simulink model "Pendulum_CAD_Control2293_LoopShaping_2018A"  (R2018a)
settings: Solver=ode15s  StartTime=0.0  StopTime=30  MaxStep=1e-3  RelTol=1e-3  EnableMultiTasking=on
PreLoadFcn:
  | RotaryPendulum_PARAM
values from neighbouring files (symbols this model uses):
  Kl1 = 1/db2mag(40)    [CalculoParametrosV2.m]
  Kl2 = 1/db2mag(-12)    [CalculoParametrosV2.m]
  s = tf('s')    [CalculoParametrosV2.m]
undefined symbols (not defined in the file or in its folder): controller_on_off, K2, length_base, length_vert_cylinder, radius_vert_cylinder, X, Y, Z
libraries: sm_lib x48, nesl_utility x6, fl_lib x4, cstblocks x2, simulink x1, aerolibanimutils x1
(part 1 of 2)
settings Model: ParamWorkspaceSource=ReferencedWorkspace  TunableVars=controller_on_off,friction_on_off  TunableVarsStorageClass=ExportedGlobal,ExportedGlobal  TunableVarsTypeQualifier=,  Creator=smalack  LastModifiedBy=Marcelo
settings DataIOCC: LimitDataPoints=on  SaveFormat=Array
settings OptimizationCC: DefaultParameterBehavior=Inlined  LifeSpan=inf
settings DebuggingCC: SFUnexpectedBacktrackingDiag=warning  SFNoUnconditionalDefaultTransitionDiag=warning  SFExecutionAtInitializationDiag=none
settings HardwareCC: ProdBitPerPointer=32  ProdBitPerSizeT=32  ProdBitPerPtrDiffT=32  ProdLargestAtomicFloat=None  ProdIntDivRoundTo=Undefined  ProdEndianess=Unspecified  ProdWordSize=32  ProdHWDeviceType=32-bit Generic
settings ModelReferenceCC: PropagateSignalLabelsOutOfModel=off
settings CodeAppCC: StateflowObjectComments=on
settings GRTTargetCC: TargetLangStandard=C89/C90 (ANSI)
settings ConfigComp: CovMetricSettings=dw  CovHtmlReporting=on  CovSaveCumulativeToWorkspaceVar=on  CovSaveSingleToWorkspaceVar=on  CovExternalEMLEnable=off
settings SimscapeCC: SimscapeNormalizeSystem=off
settings ConfigurationSet: Description=SimMechanics 2G
settings ExplorerConfigSet: InternalSimMechanicsExplorerSettings="<ExplorerConfiguration><canonicalview>default</canonicalview><AnimationSetting><BasePlaybackSpeed>1.0</BasePlaybackSpeed><PlaybackSpeedFactor>1.0</PlaybackSpeedFactor></AnimationSetting><TilePanel><TileInfo><Tiles Columns=\"1\" Count=\"1\" Rows=\"1\"><Column Weight=\"1\"/><Row Weight=\"1\"/><Tile Height=\"1\" Width=\"1\" X=\"0\" Y=\"0\"/></Tiles></TileInfo><SceneInfo><SceneViewer><BGColor><R>0.866666674613952637</R><G>0.866666674613952637</G><B>0.866666674613952637</B></BGColor><Camera><DoPerspective>off</DoPerspective><Position><X>0.54567988539648471</X><Y>0.116966334833298546</Y><Z>0.211463718228743575</Z></Position><Center><X>0.0539563667929072593</X><Y>0.0515860641109495213</Y><Z>0.183072620253275059</Z></Center><Up><X>-0.0571571554031080065</X><Y>-0.00365517739132248387</Y><Z>0.998358502375005452</Z></Up><ViewLimDist>1</ViewLimDist><YLim>0.200635310715059134</YLim><XLim>0.295379762997170392</XLim></Camera></SceneViewer></SceneInfo></TilePanel><MechEditorPanel><Cameras/><GfxPanelCameraMap/><VideoCreator><PlaybackSpeedRatio>1.0</PlaybackSpeedRatio><FrameRate>30</FrameRate><VideoFormat>MPEG-4</VideoFormat><FrameSize>auto</FrameSize></VideoCreator></MechEditorPanel></ExplorerConfiguration>"

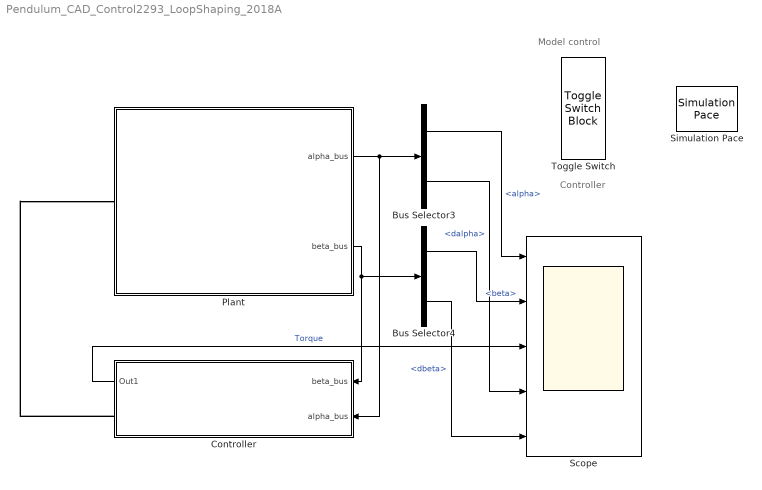
== system Pendulum_CAD_Control2293_LoopShaping_2018A ==
  note: Model control
  note: Controller
  Bus Selector3 : BusSelector  OutputSignals=alpha,dalpha
  Bus Selector4 : BusSelector  OutputSignals=beta,dbeta
  Controller : Subsystem  mask{energy_gain=0.36, switch_angle=30, alpha=K2(1), alpha_dot=K2(3), beta=K2(2), beta_dot=K2(4)}
      mask prompts: energy_gain "energy control gain [-]"; switch_angle "switch angle [deg]"; alpha "alpha [-]"; alpha_dot "alpha_dot [-]"; beta "beta [-]"; beta_dot "beta_dot [-]"
      mask DialogControl Container20 Prompt: SwingUp Control
      mask DialogControl Container17 Prompt: SwingUp to StayUp
      mask DialogControl Container10 Prompt: StayUp Control
      mask Display:
      | disp('{\itcontrol variable=}  k\timesE\timessign(\partial{\beta}/\partial{t} \times cos(\beta))', 'texmode','on')
      | port_label('input', 2, 'alpha_bus')
      | port_label('input', 1, 'beta_bus')
  Plant : Subsystem
      mask Display:
      | image('overall.JPG')
      | port_label('lconn',1,'torque');
      | port_label('output', 1, 'alpha_bus')
      | port_label('output', 2, 'beta_bus')
  Scope : Scope  NumInputPorts=5
  Simulation Pace : aerolibanimutils/Simulation Pace  SimulationPace=1  SleepMode=MATLAB Thread  OutputPaceError=off  SampleTime=1/30
      settings: AttributesFormatString=%<SimulationPace> sec/sec
  Toggle Switch : ToggleSwitchBlock  WebBlockId=671
      settings: Values={{'Off', 'On'}, [0 1]}
  wires:
  Plant/2(beta_bus) -> Controller/1(beta_bus), Bus Selector4/1
  Plant/1(alpha_bus) -> Bus Selector3/1, Controller/2(alpha_bus)
  Bus Selector3/1 -> Scope/1  "<alpha>"
  Bus Selector4/1 -> Scope/2  "<beta>"
  Bus Selector3/2 -> Scope/4  "<dalpha>"
  Bus Selector4/2 -> Scope/5  "<dbeta>"
  Controller/1(Out1) -> Scope/3  "Torque"
  connections:
  Controller/RConn1 -- Plant/LConn1

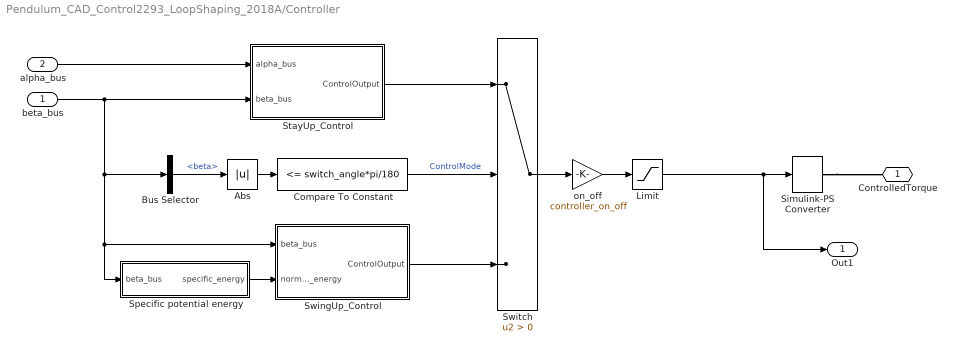
== system Pendulum_CAD_Control2293_LoopShaping_2018A/Controller ==
  beta_bus : Inport
  alpha_bus : Inport  Port=2
  Abs : Abs
  Bus Selector : BusSelector  OutputSignals=beta
  Compare To Constant : simulink/Logic and Bit Operations/Compare To Constant  relop=<=  const=switch_angle*pi/180  OutDataTypeStr=boolean
  Limit : Saturate  UpperLimit=0.1e3  LowerLimit=-0.1e3
  Simulink-PS Converter : nesl_utility/Simulink-PS Converter  PhysicalDomain=network_engine_domain  SubClassName=ps_input  LeftPortType=input  RightPortType=output  PseudoPeriodic=off  Frequencies=[]  NoiseDistribution=none  NoiseParameters=[]  Unit=N*mm  AffineConversion=off  FilteringAndDerivatives=zero  SimscapeFilterOrder=1  InputFilterTimeConstant=0.001  UdotUserProvided=1
  Specific potential energy : Subsystem
  StayUp_Control : Subsystem
  SwingUp_Control : Subsystem  mask{Gain=energy_gain}
      mask prompts: Gain "Simulink:blkprm_prompts:GainGain"
      mask TypeOptions Gain: Gain/Gain
      mask DialogControl Gain Prompt: Gain:
  Switch : Switch  Criteria=u2 > Threshold
  on_off : Gain  Gain=controller_on_off
  ControlledTorque : PMIOPort  Side=Right
  Out1 : Outport  VectorParamsAs1DForOutWhenUnconnected=off
  wires:
  alpha_bus/1 -> StayUp_Control/1(alpha_bus)
  Compare To Constant/1 -> Switch/2  "ControlMode"
  Abs/1 -> Compare To Constant/1
  Bus Selector/1 -> Abs/1  "<beta>"
  beta_bus/1 -> StayUp_Control/2(beta_bus), SwingUp_Control/1(beta_bus), Specific potential energy/1(beta_bus), Bus Selector/1
  SwingUp_Control/1(ControlOutput) -> Switch/3
  Switch/1 -> on_off/1
  on_off/1 -> Limit/1
  Specific potential energy/1(specific_energy) -> SwingUp_Control/2(normalized_energy)
  Limit/1 -> Out1/1, Simulink-PS Converter/1
  StayUp_Control/1(ControlOutput) -> Switch/1
  connections:
  Simulink-PS Converter/RConn1 -- ControlledTorque/RConn1

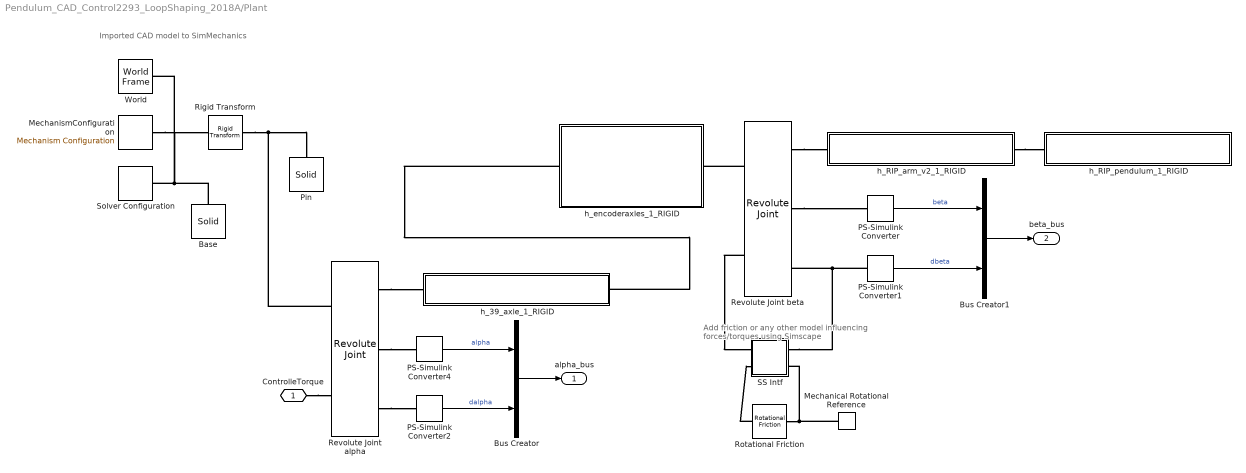
== system Pendulum_CAD_Control2293_LoopShaping_2018A/Plant ==
  note: Imported CAD model to SimMechanics
  note: Add friction or any other model
      | influencing forces/torques using Simscape
  Base : sm_lib/Body Elements/Solid  GraphicAmbientColor=[0.15 0.15 0.15 1.0]  BasedOnType=Density  CenterOfMass=[0 0 0]  CenterOfMassUnits=m  GraphicDiffuseColor=[0.4 0.4 0.4]  CylinderLength=length_base  CylinderLengthUnits=m  CylinderRadius=radius_base  CylinderRadiusUnits=m  Density=2700  DensityUnits=kg/(m^3)  DoExposeReferenceFrame=on  GraphicEmissiveColor=[0.0 0.0 0.0 1.0]  ExportEntireGeometry=off  SerializedFrames=<Frames/>  MarkerShape=Sphere  MarkerSize=10  GraphicType=FromGeometry  InertiaType=CalculateFromGeometry  Mass=1  MassUnits=kg  MomentsOfInertia=[1 1 1]  MomentsOfInertiaUnits=kg*m^2  GraphicOpacity=1.0  ProductsOfInertia=[0 0 0]  ProductsOfInertiaUnits=kg*m^2  GraphicShininess=75  GraphicSpecularColor=[0.5 0.5 0.5 1.0]  GraphicVisPropType=SimpleVisualProperties  GeometryShape=Cylinder
  Bus Creator : BusCreator  Inputs=2
  Bus Creator1 : BusCreator  Inputs=2
  Mechanical Rotational Reference : fl_lib/Mechanical/Rotational Elements/Mechanical Rotational Reference
  MechanismConfiguration : sm_lib/Utilities/Mechanism Configuration  UniformGravity=Constant  GravityVector=[0 0 -9.81]  GravityUnits=m/s^2  LinearizationDelta=0.001
  PS-Simulink Converter : nesl_utility/PS-Simulink Converter  PhysicalDomain=network_engine_domain  SubClassName=ps_output  LeftPortType=input  RightPortType=output  PseudoPeriodic=off  Frequencies=[]  Unit=rad  AffineConversion=off
  PS-Simulink Converter1 : nesl_utility/PS-Simulink Converter  PhysicalDomain=network_engine_domain  SubClassName=ps_output  LeftPortType=input  RightPortType=output  PseudoPeriodic=off  Frequencies=[]  Unit=rad/s  AffineConversion=off
  PS-Simulink Converter2 : nesl_utility/PS-Simulink Converter  PhysicalDomain=network_engine_domain  SubClassName=ps_output  LeftPortType=input  RightPortType=output  PseudoPeriodic=off  Frequencies=[]  Unit=rad/s  AffineConversion=off
  PS-Simulink Converter4 : nesl_utility/PS-Simulink Converter  PhysicalDomain=network_engine_domain  SubClassName=ps_output  LeftPortType=input  RightPortType=output  PseudoPeriodic=off  Frequencies=[]  Unit=rad  AffineConversion=off
  Pin : sm_lib/Body Elements/Solid  GraphicAmbientColor=[0.15 0.15 0.15 1.0]  BasedOnType=Density  CenterOfMass=[0 0 0]  CenterOfMassUnits=m  GraphicDiffuseColor=[0.8 0.6 1.0]  CylinderLength=length_vert_cylinder  CylinderLengthUnits=m  CylinderRadius=radius_vert_cylinder/2  CylinderRadiusUnits=m  Density=2700  DensityUnits=kg/(m^3)  DoExposeReferenceFrame=on  GraphicEmissiveColor=[0.0 0.0 0.0 1.0]  ExportEntireGeometry=off  SerializedFrames=<Frames/>  MarkerShape=Sphere  MarkerSize=10  GraphicType=FromGeometry  InertiaType=CalculateFromGeometry  Mass=1  MassUnits=kg  MomentsOfInertia=[1 1 1]  MomentsOfInertiaUnits=kg*m^2  GraphicOpacity=.5  ProductsOfInertia=[0 0 0]  ProductsOfInertiaUnits=kg*m^2  GraphicShininess=75  GraphicSpecularColor=[0.5 0.5 0.5 1.0]  GraphicVisPropType=SimpleVisualProperties  GeometryShape=Cylinder
  Revolute Joint alpha : sm_lib/Joints/Revolute Joint  JointMode=Normal  SenseConstraintForce=off  SenseConstraintForceX=off  SenseConstraintForceY=off  SenseConstraintForceZ=off  SenseConstraintTorque=off  SenseConstraintTorqueX=off  SenseConstraintTorqueY=off  SenseConstraintTorqueZ=off  SenseTotalForce=off  SenseTotalForceX=off  SenseTotalForceY=off  SenseTotalForceZ=off  SenseTotalTorque=off  SenseTotalTorqueX=off  SenseTotalTorqueY=off  SenseTotalTorqueZ=off  CompositeWrenchDir=FollowerOnBase  CompositeWrenchFrame=BaseFrame  EquilibriumPosition=0  EquilibriumPositionUnits=deg  SpringStiffness=1e-7  SpringStiffnessUnits=N*m/deg  DampingCoefficient=1e-6  DampingCoefficientUnits=N*m/(deg/s)  TorqueActuationMode=InputTorque  MotionActuationMode=ComputedMotion  SensePosition=on  SenseVelocity=on  SenseAcceleration=off  SenseTorqueForce=off  SenseLowerLimitTorqueForce=off  SenseUpperLimitTorqueForce=off  LowerLimitSpecify=off  LowerLimitBound=-90  LowerLimitBoundUnits=deg  LowerLimitStiffness=1e4  LowerLimitStiffnessUnits=N*m/deg  LowerLimitDamping=10  LowerLimitDampingUnits=N*m/(deg/s)  LowerLimitTransitionRegionWidth=0.1  LowerLimitTransitionRegionWidthUnits=deg  UpperLimitSpecify=off  UpperLimitBound=90  UpperLimitBoundUnits=deg  UpperLimitStiffness=1e4  UpperLimitStiffnessUnits=N*m/deg  UpperLimitDamping=10  UpperLimitDampingUnits=N*m/(deg/s)  UpperLimitTransitionRegionWidth=0.1  UpperLimitTransitionRegionWidthUnits=deg  PositionTargetSpecify=off  PositionTargetPriority=High  PositionTargetValue=pi  PositionTargetValueUnits=rad  VelocityTargetSpecify=off  VelocityTargetPriority=High  VelocityTargetValue=0  VelocityTargetValueUnits=deg/s
  Revolute Joint beta : sm_lib/Joints/Revolute Joint  JointMode=Normal  SenseConstraintForce=off  SenseConstraintForceX=off  SenseConstraintForceY=off  SenseConstraintForceZ=off  SenseConstraintTorque=off  SenseConstraintTorqueX=off  SenseConstraintTorqueY=off  SenseConstraintTorqueZ=off  SenseTotalForce=off  SenseTotalForceX=off  SenseTotalForceY=off  SenseTotalForceZ=off  SenseTotalTorque=off  SenseTotalTorqueX=off  SenseTotalTorqueY=off  SenseTotalTorqueZ=off  CompositeWrenchDir=FollowerOnBase  CompositeWrenchFrame=BaseFrame  EquilibriumPosition=0  EquilibriumPositionUnits=rad  SpringStiffness=0  SpringStiffnessUnits=m*N/rad  DampingCoefficient=0  DampingCoefficientUnits=m*s*N/rad  TorqueActuationMode=InputTorque  MotionActuationMode=ComputedMotion  SensePosition=on  SenseVelocity=on  SenseAcceleration=off  SenseTorqueForce=off  SenseLowerLimitTorqueForce=off  SenseUpperLimitTorqueForce=off  LowerLimitSpecify=off  LowerLimitBound=-90  LowerLimitBoundUnits=deg  LowerLimitStiffness=1e4  LowerLimitStiffnessUnits=N*m/deg  LowerLimitDamping=10  LowerLimitDampingUnits=N*m/(deg/s)  LowerLimitTransitionRegionWidth=0.1  LowerLimitTransitionRegionWidthUnits=deg  UpperLimitSpecify=off  UpperLimitBound=90  UpperLimitBoundUnits=deg  UpperLimitStiffness=1e4  UpperLimitStiffnessUnits=N*m/deg  UpperLimitDamping=10  UpperLimitDampingUnits=N*m/(deg/s)  UpperLimitTransitionRegionWidth=0.1  UpperLimitTransitionRegionWidthUnits=deg  PositionTargetSpecify=on  PositionTargetPriority=Low  PositionTargetValue=180  PositionTargetValueUnits=deg  VelocityTargetSpecify=on  VelocityTargetPriority=High  VelocityTargetValue=0  VelocityTargetValueUnits=deg/s
  Rigid Transform : sm_lib/Frames and Transforms/Rigid Transform  TranslationMethod=StandardAxis  TranslationStandardOffset=length_base/2+length_vert_cylinder/2  TranslationLengthUnit=m  TranslationStandardAxis=+Z  TranslationCartesianOffset=[0 0 0]  TranslationROffset=0  TranslationROffsetUnits=m  TranslationZOffset=0  TranslationZOffsetUnits=m  TranslationThetaOffset=0  TranslationThetaOffsetUnits=deg  RotationMethod=None  RotationAngleUnits=deg  RotationStandardAxis=+Z  RotationAngle=0.0  RotationArbitraryAxis=[0 0 1]  FollAlignAxisA=+X  BaseAlignAxisA=+Y  FollAlignAxisB=+Y  BaseAlignAxisB=+Z  RotationSequenceAxes=FollowerAxes  RotationSequence=XYX  RotationSequenceAngles=[0 0 0]  RotationSequenceAnglesUnits=deg  RotationMatrix=[1 0 0; 0 1 0; 0 0 1]
  Rotational Friction : fl_lib/Mechanical/Rotational Elements/Rotational Friction  brkwy_trq=0.0004 mN*m  brkwy_vel=0.12128 rad/s  Col_trq=0.0002 mN*m  visc_coef=0.001 m*s*mN/rad  w_specify=off  w_priority=High  w=0 rad/s  w_nominal_specify=off  w_nominal_unit=rad/s  w_nominal_value=1  t_specify=off  t_priority=High  t=0 N*m  t_nominal_specify=off  t_nominal_unit=N*m  t_nominal_value=1
  SS Intf : Subsystem
  Solver Configuration : nesl_utility/Solver Configuration  PhysicalDomain=network_engine_domain  SubClassName=solver  LeftPortType=input  RightPortType=generic  Tones=[]  Harmonics=[]  SimulateNoise=off  Profile=off  UseLocalSampling=off  EnableSwitchedLinearOptims=on  FrequencyDomain=off  UseCCode=off  RelTol=0.001  AbsTol=1e-06  MinStep=1e-09  ToWorkspace=off  RevertToSquareIcSolve=off  NumHomotopyIterations=100  PhasorMode=off  PhasorModeNumHarmonics=1  DoDC=off  ResidualTolerance=1e-09  UseLocalSolver=off  LocalSolverChoice=NE_BACKWARD_EULER_ADVANCER  LocalSolverSampleTime=1e-3  DoFixedCost=off  MaxNonlinIter=3  MaxModeIter=2  LinearAlgebra=Sparse  EquationFormulation=NE_TIME_EF  DelaysMemoryBudget=1024  AutomaticFiltering=on  FilteringTimeConstant=0.001  PartitionStorageMethod=AS_NEEDED  PartitionMemoryBudget=1024  PartitionMethod=FAST
  World : sm_lib/Frames and Transforms/World Frame
  h_39_axle_1_RIGID : Subsystem
      mask Display:
      | image('h_39_axle_1_RIGID.JPG')
      | port_label('lconn',1,'B');
      | port_label('rconn',1,'R');
  h_RIP_arm_v2_1_RIGID : Subsystem
      mask Display:
      | image('h_RIP_arm_v2_1_RIGID.JPG');
      | port_label('lconn',1,'B');
      | port_label('rconn',1,'R');
  h_RIP_pendulum_1_RIGID : Subsystem
      mask Display: image('h_RIP_pendulum_1_RIGID.JPG');
  h_encoderaxles_1_RIGID : Subsystem
      mask Display:
      | image('h_encoderaxles_1_RIGID.JPG');
      | port_label('lconn',1,'B');
      | port_label('rconn',1,'R');
  ControlleTorque : PMIOPort  Side=Left
  alpha_bus : Outport  VectorParamsAs1DForOutWhenUnconnected=off
  beta_bus : Outport  Port=2  VectorParamsAs1DForOutWhenUnconnected=off
  wires:
  Bus Creator/1 -> alpha_bus/1
  Bus Creator1/1 -> beta_bus/1
  PS-Simulink Converter/1 -> Bus Creator1/1  "beta"
  PS-Simulink Converter4/1 -> Bus Creator/1  "alpha"
  PS-Simulink Converter2/1 -> Bus Creator/2  "dalpha"
  PS-Simulink Converter1/1 -> Bus Creator1/2  "dbeta"
  connections:
  Rotational Friction/LConn1 -- SS Intf/RConn2
  Revolute Joint beta/RConn1 -- h_RIP_arm_v2_1_RIGID/LConn1
  Rotational Friction/RConn1 -- Mechanical Rotational Reference/LConn1 -- SS Intf/LConn2
  Revolute Joint alpha/RConn1 -- h_39_axle_1_RIGID/LConn1
  PS-Simulink Converter1/LConn1 -- SS Intf/LConn1 -- Revolute Joint beta/RConn3
  Base/RConn1 -- Rigid Transform/LConn1 -- MechanismConfiguration/RConn1 -- World/RConn1 -- Solver Configuration/RConn1
  Revolute Joint alpha/RConn3 -- PS-Simulink Converter2/LConn1
  h_encoderaxles_1_RIGID/LConn1 -- h_39_axle_1_RIGID/RConn1
  h_RIP_arm_v2_1_RIGID/RConn1 -- h_RIP_pendulum_1_RIGID/LConn1
  Revolute Joint beta/LConn1 -- h_encoderaxles_1_RIGID/RConn1
  Revolute Joint beta/LConn2 -- SS Intf/RConn1
  Revolute Joint alpha/RConn2 -- PS-Simulink Converter4/LConn1
  Revolute Joint beta/RConn2 -- PS-Simulink Converter/LConn1
  ControlleTorque/RConn1 -- Revolute Joint alpha/LConn2
  Rigid Transform/RConn1 -- Revolute Joint alpha/LConn1 -- Pin/RConn1

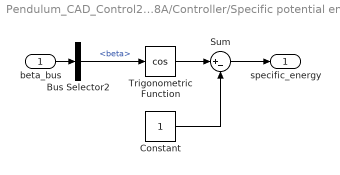
== system Pendulum_CAD_Control2293_LoopShaping_2018A/Controller/Specific potential energy ==
  beta_bus : Inport
  Bus Selector2 : BusSelector  OutputSignals=beta
  Constant : Constant
  Sum : Sum  Inputs=|+-
  Trigonometric Function : Trigonometry  Operator=cos
  specific_energy : Outport  VectorParamsAs1DForOutWhenUnconnected=off
  wires:
  Constant/1 -> Sum/2
  Trigonometric Function/1 -> Sum/1
  Sum/1 -> specific_energy/1
  Bus Selector2/1 -> Trigonometric Function/1  "<beta>"
  beta_bus/1 -> Bus Selector2/1

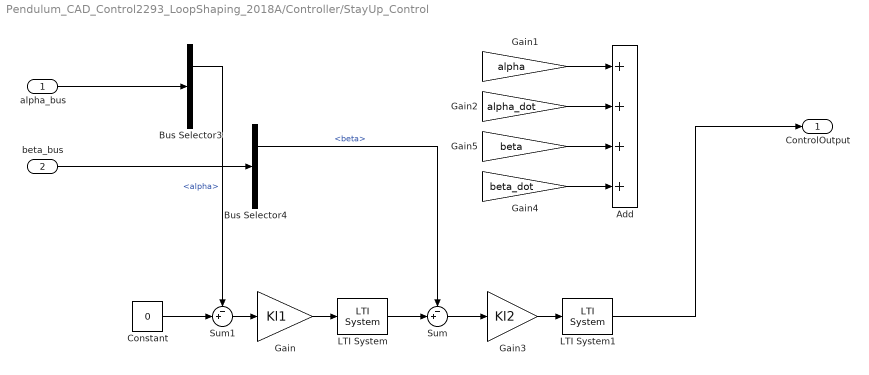
== system Pendulum_CAD_Control2293_LoopShaping_2018A/Controller/StayUp_Control ==
  alpha_bus : Inport
  beta_bus : Inport  Port=2
  Add : Sum  Inputs=++++
  Bus Selector3 : BusSelector  OutputSignals=alpha,dalpha
  Bus Selector4 : BusSelector  OutputSignals=beta,dbeta
  Constant : Constant  Value=0
  Gain : Gain  Gain=Kl1
  Gain1 : Gain  Gain=alpha
  Gain2 : Gain  Gain=alpha_dot
  Gain3 : Gain  Gain=Kl2
  Gain4 : Gain  Gain=beta_dot
  Gain5 : Gain  Gain=beta
  LTI System : cstblocks/LTI System  sys=C1  IC=[]
  LTI System1 : cstblocks/LTI System  sys=C2  IC=[]
  Sum : Sum  Inputs=-+|
  Sum1 : Sum  Inputs=-+|
  ControlOutput : Outport  VectorParamsAs1DForOutWhenUnconnected=off
  wires:
  alpha_bus/1 -> Bus Selector3/1
  Gain5/1 -> Add/3
  Gain1/1 -> Add/1
  Gain4/1 -> Add/4
  beta_bus/1 -> Bus Selector4/1
  Gain2/1 -> Add/2
  Bus Selector3/1 -> Sum1/1  "<alpha>"
  Constant/1 -> Sum1/2
  LTI System1/1 -> ControlOutput/1
  Gain/1 -> LTI System/1
  Sum1/1 -> Gain/1
  Gain3/1 -> LTI System1/1
  Sum/1 -> Gain3/1
  Bus Selector4/1 -> Sum/1  "<beta>"
  LTI System/1 -> Sum/2

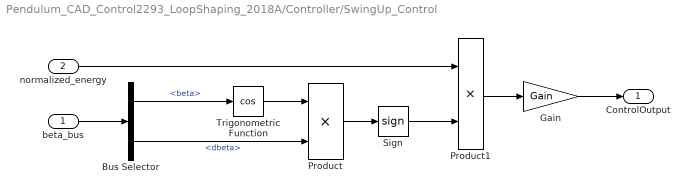
== system Pendulum_CAD_Control2293_LoopShaping_2018A/Controller/SwingUp_Control ==
  beta_bus : Inport
  normalized_energy : Inport  Port=2
  Bus Selector : BusSelector  OutputSignals=beta,dbeta
  Gain : Gain  Gain=Gain
  Product : Product
  Product1 : Product
  Sign : Signum
  Trigonometric Function : Trigonometry  Operator=cos
  ControlOutput : Outport  VectorParamsAs1DForOutWhenUnconnected=off
  wires:
  Product/1 -> Sign/1
  Trigonometric Function/1 -> Product/1
  Gain/1 -> ControlOutput/1
  Sign/1 -> Product1/2
  Product1/1 -> Gain/1
  normalized_energy/1 -> Product1/1
  beta_bus/1 -> Bus Selector/1
  Bus Selector/1 -> Trigonometric Function/1  "<beta>"
  Bus Selector/2 -> Product/2  "<dbeta>"

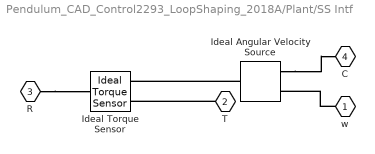
== system Pendulum_CAD_Control2293_LoopShaping_2018A/Plant/SS Intf ==
  Ideal Angular Velocity Source : fl_lib/Mechanical/Mechanical Sources/Ideal Angular Velocity Source
  Ideal Torque Sensor : fl_lib/Mechanical/Mechanical Sensors/Ideal Torque Sensor
  w : PMIOPort  Side=Left
  T : PMIOPort  Port=2  Side=Right
  R : PMIOPort  Port=3  Side=Right
  C : PMIOPort  Port=4  Side=Left
  connections:
  w/RConn1 -- Ideal Angular Velocity Source/RConn1
  R/RConn1 -- Ideal Torque Sensor/LConn1
  Ideal Angular Velocity Source/RConn2 -- C/RConn1
  Ideal Angular Velocity Source/LConn1 -- Ideal Torque Sensor/RConn1
  T/RConn1 -- Ideal Torque Sensor/RConn2

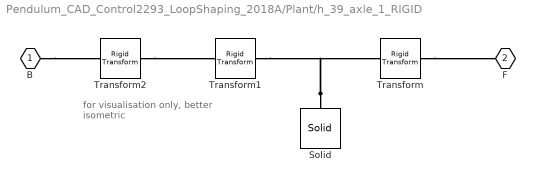
== system Pendulum_CAD_Control2293_LoopShaping_2018A/Plant/h_39_axle_1_RIGID ==
  note: for visualisation only,
      | better isometric
  Solid : sm_lib/Body Elements/Solid  ExtGeomFileName=h_39_axle_Default_sldprt.STL  UnitType=Custom  ExtGeomFileUnits=mm  StepReaderType=HEX  ExportConvexHullGeometry=off  InertiaType=Custom  Mass=0.00052672018519800228  MassUnits=kg  CenterOfMass=[0 0 0]  CenterOfMassUnits=mm  MomentsOfInertia=[0.0012508560304239273 0.066771141817072402 0.066771141817072402]  MomentsOfInertiaUnits=kg*mm^2  ProductsOfInertia=[0 0 0]  ProductsOfInertiaUnits=kg*mm^2  BasedOnType=Density  Density=1000  DensityUnits=kg/(m^3)  DoExposeReferenceFrame=on  SerializedFrames=<Frames/>  GraphicType=FromGeometry  MarkerShape=Sphere  MarkerSize=10  MarkerSizeUnits=m  GraphicVisPropType=SimpleVisualProperties  GraphicDiffuseColor=[0.4 0.4 0.4]  GraphicSpecularColor=[0.5 0.5 0.5 1.0]  GraphicAmbientColor=[0.15 0.15 0.15 1.0]  GraphicEmissiveColor=[0.0 0.0 0.0 1.0]  GraphicShininess=75  GraphicOpacity=1  GeometryShape=FromFile
  Transform : sm_lib/Frames and Transforms/Rigid Transform  TranslationMethod=Cartesian  TranslationStandardOffset=0  TranslationLengthUnit=mm  TranslationStandardAxis=+Z  TranslationCartesianOffset=[19.5 1.2534832698893993 1.25543121904946712 ]  TranslationROffset=0  TranslationROffsetUnits=m  TranslationZOffset=0  TranslationZOffsetUnits=m  TranslationThetaOffset=0  TranslationThetaOffsetUnits=deg  RotationMethod=StandardAxis  RotationAngleUnits=rad  RotationStandardAxis=-Y  RotationAngle=pi/2  RotationArbitraryAxis=[0.70549464967288755 0.067487766045881178 -0.70549464967288456]  FollAlignAxisA=+X  BaseAlignAxisA=+Y  FollAlignAxisB=+Y  BaseAlignAxisB=+Z  RotationSequenceAxes=FollowerAxes  RotationSequence=XYX  RotationSequenceAngles=[0 0 0]  RotationSequenceAnglesUnits=deg  RotationMatrix=[1 0 0; 0 1 0; 0 0 1]
  Transform1 : sm_lib/Frames and Transforms/Rigid Transform  TranslationMethod=Cartesian  TranslationStandardOffset=0  TranslationLengthUnit=mm  TranslationStandardAxis=+Z  TranslationCartesianOffset=[0 0 19.5]  TranslationROffset=0  TranslationROffsetUnits=m  TranslationZOffset=0  TranslationZOffsetUnits=m  TranslationThetaOffset=0  TranslationThetaOffsetUnits=deg  RotationMethod=StandardAxis  RotationAngleUnits=rad  RotationStandardAxis=-Y  RotationAngle=pi/2  RotationArbitraryAxis=[0.70549464967288755 0.067487766045881178 -0.70549464967288456]  FollAlignAxisA=+X  BaseAlignAxisA=+Y  FollAlignAxisB=+Y  BaseAlignAxisB=+Z  RotationSequenceAxes=FollowerAxes  RotationSequence=XYX  RotationSequenceAngles=[0 0 0]  RotationSequenceAnglesUnits=deg  RotationMatrix=[1 0 0; 0 1 0; 0 0 1]
  Transform2 : sm_lib/Frames and Transforms/Rigid Transform  TranslationMethod=Cartesian  TranslationStandardOffset=0  TranslationLengthUnit=mm  TranslationStandardAxis=+Z  TranslationCartesianOffset=[0 0 19.5]  TranslationROffset=0  TranslationROffsetUnits=m  TranslationZOffset=0  TranslationZOffsetUnits=m  TranslationThetaOffset=0  TranslationThetaOffsetUnits=deg  RotationMethod=StandardAxis  RotationAngleUnits=rad  RotationStandardAxis=+Z  RotationAngle=pi  RotationArbitraryAxis=[0.70549464967288755 0.067487766045881178 -0.70549464967288456]  FollAlignAxisA=+X  BaseAlignAxisA=+Y  FollAlignAxisB=+Y  BaseAlignAxisB=+Z  RotationSequenceAxes=FollowerAxes  RotationSequence=XYX  RotationSequenceAngles=[0 0 0]  RotationSequenceAnglesUnits=deg  RotationMatrix=[1 0 0; 0 1 0; 0 0 1]
  B : PMIOPort  Side=Left
  F : PMIOPort  Port=2  Side=Right
  connections:
  Solid/RConn1 -- Transform1/RConn1 -- Transform/LConn1
  Transform/RConn1 -- F/RConn1
  Transform2/RConn1 -- Transform1/LConn1
  B/RConn1 -- Transform2/LConn1

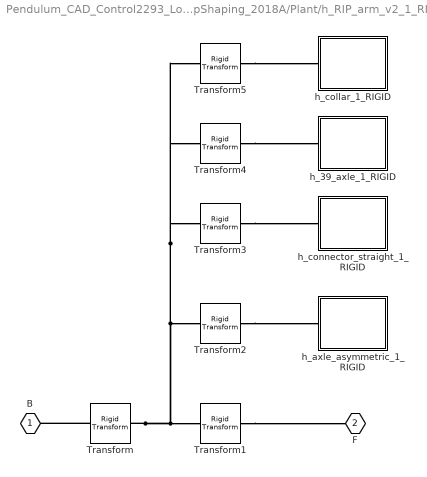
== system Pendulum_CAD_Control2293_LoopShaping_2018A/Plant/h_RIP_arm_v2_1_RIGID ==
  Transform : sm_lib/Frames and Transforms/Rigid Transform  TranslationMethod=Cartesian  TranslationStandardOffset=0  TranslationLengthUnit=mm  TranslationStandardAxis=+Z  TranslationCartesianOffset=[-2.3499999999999996 11.000000000000007 49.543413938003653]  TranslationROffset=0  TranslationROffsetUnits=m  TranslationZOffset=0  TranslationZOffsetUnits=m  TranslationThetaOffset=0  TranslationThetaOffsetUnits=deg  RotationMethod=ArbitraryAxis  RotationAngleUnits=rad  RotationStandardAxis=+Z  RotationAngle=2.0943951023931953  RotationArbitraryAxis=[0.57735026918962584 -0.57735026918962595 0.57735026918962562]  FollAlignAxisA=+X  BaseAlignAxisA=+Y  FollAlignAxisB=+Y  BaseAlignAxisB=+Z  RotationSequenceAxes=FollowerAxes  RotationSequence=XYX  RotationSequenceAngles=[0 0 0]  RotationSequenceAnglesUnits=deg  RotationMatrix=[1 0 0; 0 1 0; 0 0 1]
  Transform1 : sm_lib/Frames and Transforms/Rigid Transform  TranslationMethod=Cartesian  TranslationStandardOffset=0  TranslationLengthUnit=mm  TranslationStandardAxis=+Z  TranslationCartesianOffset=[52.337380238255371 20.27500000000154 24.811029445672951]  TranslationROffset=0  TranslationROffsetUnits=m  TranslationZOffset=0  TranslationZOffsetUnits=m  TranslationThetaOffset=0  TranslationThetaOffsetUnits=deg  RotationMethod=ArbitraryAxis  RotationAngleUnits=rad  RotationStandardAxis=+Z  RotationAngle=2.0943951023931953  RotationArbitraryAxis=[-0.57735026918962562 -0.57735026918962584 -0.57735026918962584]  FollAlignAxisA=+X  BaseAlignAxisA=+Y  FollAlignAxisB=+Y  BaseAlignAxisB=+Z  RotationSequenceAxes=FollowerAxes  RotationSequence=XYX  RotationSequenceAngles=[0 0 0]  RotationSequenceAnglesUnits=deg  RotationMatrix=[1 0 0; 0 1 0; 0 0 1]
  Transform2 : sm_lib/Frames and Transforms/Rigid Transform  TranslationMethod=Cartesian  TranslationStandardOffset=0  TranslationLengthUnit=mm  TranslationStandardAxis=+Z  TranslationCartesianOffset=[-2.3499999999999908 64.5 49.543413938003681]  TranslationROffset=0  TranslationROffsetUnits=m  TranslationZOffset=0  TranslationZOffsetUnits=m  TranslationThetaOffset=0  TranslationThetaOffsetUnits=deg  RotationMethod=ArbitraryAxis  RotationAngleUnits=rad  RotationStandardAxis=+Z  RotationAngle=1.5707963267948966  RotationArbitraryAxis=[0 0 1]  FollAlignAxisA=+X  BaseAlignAxisA=+Y  FollAlignAxisB=+Y  BaseAlignAxisB=+Z  RotationSequenceAxes=FollowerAxes  RotationSequence=XYX  RotationSequenceAngles=[0 0 0]  RotationSequenceAnglesUnits=deg  RotationMatrix=[1 0 0; 0 1 0; 0 0 1]
  Transform3 : sm_lib/Frames and Transforms/Rigid Transform  TranslationMethod=Cartesian  TranslationStandardOffset=0  TranslationLengthUnit=mm  TranslationStandardAxis=+Z  TranslationCartesianOffset=[-2.3499999999999908 56.699999999999996 49.543413938003681]  TranslationROffset=0  TranslationROffsetUnits=m  TranslationZOffset=0  TranslationZOffsetUnits=m  TranslationThetaOffset=0  TranslationThetaOffsetUnits=deg  RotationMethod=ArbitraryAxis  RotationAngleUnits=rad  RotationStandardAxis=+Z  RotationAngle=1.5707963267948966  RotationArbitraryAxis=[0 0 1]  FollAlignAxisA=+X  BaseAlignAxisA=+Y  FollAlignAxisB=+Y  BaseAlignAxisB=+Z  RotationSequenceAxes=FollowerAxes  RotationSequence=XYX  RotationSequenceAngles=[0 0 0]  RotationSequenceAnglesUnits=deg  RotationMatrix=[1 0 0; 0 1 0; 0 0 1]
  Transform4 : sm_lib/Frames and Transforms/Rigid Transform  TranslationMethod=Cartesian  TranslationStandardOffset=0  TranslationLengthUnit=mm  TranslationStandardAxis=+Z  TranslationCartesianOffset=[-2.3499999999999841 84.40000000000002 49.543413938003681]  TranslationROffset=0  TranslationROffsetUnits=m  TranslationZOffset=0  TranslationZOffsetUnits=m  TranslationThetaOffset=0  TranslationThetaOffsetUnits=deg  RotationMethod=ArbitraryAxis  RotationAngleUnits=rad  RotationStandardAxis=+Z  RotationAngle=1.5707963267948966  RotationArbitraryAxis=[0 0 1]  FollAlignAxisA=+X  BaseAlignAxisA=+Y  FollAlignAxisB=+Y  BaseAlignAxisB=+Z  RotationSequenceAxes=FollowerAxes  RotationSequence=XYX  RotationSequenceAngles=[0 0 0]  RotationSequenceAnglesUnits=deg  RotationMatrix=[1 0 0; 0 1 0; 0 0 1]
  Transform5 : sm_lib/Frames and Transforms/Rigid Transform  TranslationMethod=Cartesian  TranslationStandardOffset=0  TranslationLengthUnit=mm  TranslationStandardAxis=+Z  TranslationCartesianOffset=[-2.3499999999999979 16.900000000000002 49.543413938003681]  TranslationROffset=0  TranslationROffsetUnits=m  TranslationZOffset=0  TranslationZOffsetUnits=m  TranslationThetaOffset=0  TranslationThetaOffsetUnits=deg  RotationMethod=ArbitraryAxis  RotationAngleUnits=rad  RotationStandardAxis=+Z  RotationAngle=1.5707963267948966  RotationArbitraryAxis=[0 0 1]  FollAlignAxisA=+X  BaseAlignAxisA=+Y  FollAlignAxisB=+Y  BaseAlignAxisB=+Z  RotationSequenceAxes=FollowerAxes  RotationSequence=XYX  RotationSequenceAngles=[0 0 0]  RotationSequenceAnglesUnits=deg  RotationMatrix=[1 0 0; 0 1 0; 0 0 1]
  h_39_axle_1_RIGID : Subsystem
      mask Display: image('h_39_axle_1_RIGID.JPG')
  h_axle_asymmetric_1_RIGID : Subsystem
      mask Display: image('h_axle_asymmetric_1_RIGID.JPG')
  h_collar_1_RIGID : Subsystem
      mask Display: image('h_collar_1_RIGID.JPG')
  h_connector_straight_1_RIGID : Subsystem
      mask Display: image('h_connector_straight_1_RIGID.JPG')
  B : PMIOPort  Side=Left
  F : PMIOPort  Port=2  Side=Right
  connections:
  Transform/LConn1 -- Transform1/LConn1 -- Transform2/LConn1 -- Transform3/LConn1 -- Transform4/LConn1 -- Transform5/LConn1
  Transform1/RConn1 -- F/RConn1
  Transform2/RConn1 -- h_axle_asymmetric_1_RIGID/LConn1
  Transform3/RConn1 -- h_connector_straight_1_RIGID/LConn1
  Transform4/RConn1 -- h_39_axle_1_RIGID/LConn1
  Transform5/RConn1 -- h_collar_1_RIGID/LConn1
  Transform/RConn1 -- B/RConn1

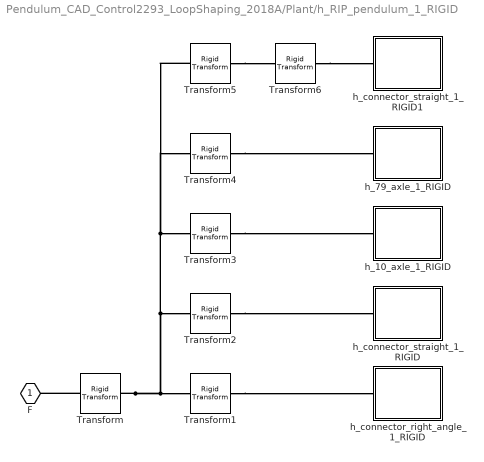
== system Pendulum_CAD_Control2293_LoopShaping_2018A/Plant/h_RIP_pendulum_1_RIGID ==
  Transform : sm_lib/Frames and Transforms/Rigid Transform  TranslationMethod=Cartesian  TranslationStandardOffset=0  TranslationLengthUnit=mm  TranslationStandardAxis=+Z  TranslationCartesianOffset=[-191.15757664014251 -77.513756526474566 -2.6766783819563784]  TranslationROffset=0  TranslationROffsetUnits=m  TranslationZOffset=0  TranslationZOffsetUnits=m  TranslationThetaOffset=0  TranslationThetaOffsetUnits=deg  RotationMethod=ArbitraryAxis  RotationAngleUnits=rad  RotationStandardAxis=+Z  RotationAngle=2.0943951023931988  RotationArbitraryAxis=[0.57735026918962673 -0.5773502691896244 0.57735026918962606]  FollAlignAxisA=+X  BaseAlignAxisA=+Y  FollAlignAxisB=+Y  BaseAlignAxisB=+Z  RotationSequenceAxes=FollowerAxes  RotationSequence=XYX  RotationSequenceAngles=[0 0 0]  RotationSequenceAnglesUnits=deg  RotationMatrix=[1 0 0; 0 1 0; 0 0 1]
  Transform1 : sm_lib/Frames and Transforms/Rigid Transform  TranslationMethod=Cartesian  TranslationStandardOffset=0  TranslationLengthUnit=mm  TranslationStandardAxis=+Z  TranslationCartesianOffset=[-136.47019640188407 -153.13875652647175 22.05570611037507]  TranslationROffset=0  TranslationROffsetUnits=m  TranslationZOffset=0  TranslationZOffsetUnits=m  TranslationThetaOffset=0  TranslationThetaOffsetUnits=deg  RotationMethod=ArbitraryAxis  RotationAngleUnits=rad  RotationStandardAxis=+Z  RotationAngle=1.5707963267948999  RotationArbitraryAxis=[0 0 1]  FollAlignAxisA=+X  BaseAlignAxisA=+Y  FollAlignAxisB=+Y  BaseAlignAxisB=+Z  RotationSequenceAxes=FollowerAxes  RotationSequence=XYX  RotationSequenceAngles=[0 0 0]  RotationSequenceAnglesUnits=deg  RotationMatrix=[1 0 0; 0 1 0; 0 0 1]
  Transform2 : sm_lib/Frames and Transforms/Rigid Transform  TranslationMethod=Cartesian  TranslationStandardOffset=0  TranslationLengthUnit=mm  TranslationStandardAxis=+Z  TranslationCartesianOffset=[-136.47019640188358 -165.03875652647181 128.15570611037563]  TranslationROffset=0  TranslationROffsetUnits=m  TranslationZOffset=0  TranslationZOffsetUnits=m  TranslationThetaOffset=0  TranslationThetaOffsetUnits=deg  RotationMethod=ArbitraryAxis  RotationAngleUnits=rad  RotationStandardAxis=+Z  RotationAngle=1.5707963267949003  RotationArbitraryAxis=[0 1 0]  FollAlignAxisA=+X  BaseAlignAxisA=+Y  FollAlignAxisB=+Y  BaseAlignAxisB=+Z  RotationSequenceAxes=FollowerAxes  RotationSequence=XYX  RotationSequenceAngles=[0 0 0]  RotationSequenceAnglesUnits=deg  RotationMatrix=[1 0 0; 0 1 0; 0 0 1]
  Transform3 : sm_lib/Frames and Transforms/Rigid Transform  TranslationMethod=Cartesian  TranslationStandardOffset=0  TranslationLengthUnit=mm  TranslationStandardAxis=+Z  TranslationCartesianOffset=[-136.47019640188373 -165.03875652647179 72.95570611037553]  TranslationROffset=0  TranslationROffsetUnits=m  TranslationZOffset=0  TranslationZOffsetUnits=m  TranslationThetaOffset=0  TranslationThetaOffsetUnits=deg  RotationMethod=ArbitraryAxis  RotationAngleUnits=rad  RotationStandardAxis=+Z  RotationAngle=1.5707963267949003  RotationArbitraryAxis=[0 1 0]  FollAlignAxisA=+X  BaseAlignAxisA=+Y  FollAlignAxisB=+Y  BaseAlignAxisB=+Z  RotationSequenceAxes=FollowerAxes  RotationSequence=XYX  RotationSequenceAngles=[0 0 0]  RotationSequenceAnglesUnits=deg  RotationMatrix=[1 0 0; 0 1 0; 0 0 1]
  Transform4 : sm_lib/Frames and Transforms/Rigid Transform  TranslationMethod=Cartesian  TranslationStandardOffset=0  TranslationLengthUnit=mm  TranslationStandardAxis=+Z  TranslationCartesianOffset=[-136.47019640188347 -165.03875652647181 159.85570611037573]  TranslationROffset=0  TranslationROffsetUnits=m  TranslationZOffset=0  TranslationZOffsetUnits=m  TranslationThetaOffset=0  TranslationThetaOffsetUnits=deg  RotationMethod=ArbitraryAxis  RotationAngleUnits=rad  RotationStandardAxis=+Z  RotationAngle=1.5707963267949003  RotationArbitraryAxis=[0 1 0]  FollAlignAxisA=+X  BaseAlignAxisA=+Y  FollAlignAxisB=+Y  BaseAlignAxisB=+Z  RotationSequenceAxes=FollowerAxes  RotationSequence=XYX  RotationSequenceAngles=[0 0 0]  RotationSequenceAnglesUnits=deg  RotationMatrix=[1 0 0; 0 1 0; 0 0 1]
  Transform5 : sm_lib/Frames and Transforms/Rigid Transform  TranslationMethod=Cartesian  TranslationStandardOffset=0  TranslationLengthUnit=mm  TranslationStandardAxis=+Z  TranslationCartesianOffset=[-136.47019640188347 -165.03875652647181 159.85570611037573]  TranslationROffset=0  TranslationROffsetUnits=m  TranslationZOffset=0  TranslationZOffsetUnits=m  TranslationThetaOffset=0  TranslationThetaOffsetUnits=deg  RotationMethod=ArbitraryAxis  RotationAngleUnits=rad  RotationStandardAxis=+Z  RotationAngle=1.5707963267949003  RotationArbitraryAxis=[0 1 0]  FollAlignAxisA=+X  BaseAlignAxisA=+Y  FollAlignAxisB=+Y  BaseAlignAxisB=+Z  RotationSequenceAxes=FollowerAxes  RotationSequence=XYX  RotationSequenceAngles=[0 0 0]  RotationSequenceAnglesUnits=deg  RotationMatrix=[1 0 0; 0 1 0; 0 0 1]
  Transform6 : sm_lib/Frames and Transforms/Rigid Transform  TranslationMethod=Cartesian  TranslationStandardOffset=0  TranslationLengthUnit=mm  TranslationStandardAxis=+Z  TranslationCartesianOffset=[-94.97019640188347/2 -0 0]  TranslationROffset=0  TranslationROffsetUnits=m  TranslationZOffset=0  TranslationZOffsetUnits=m  TranslationThetaOffset=0  TranslationThetaOffsetUnits=deg  RotationMethod=None  RotationAngleUnits=rad  RotationStandardAxis=+Z  RotationAngle=1.5707963267949003  RotationArbitraryAxis=[0 1 0]  FollAlignAxisA=+X  BaseAlignAxisA=+Y  FollAlignAxisB=+Y  BaseAlignAxisB=+Z  RotationSequenceAxes=FollowerAxes  RotationSequence=XYX  RotationSequenceAngles=[0 0 0]  RotationSequenceAnglesUnits=deg  RotationMatrix=[1 0 0; 0 1 0; 0 0 1]
  h_10_axle_1_RIGID : Subsystem
      mask Display: image('h_39_axle_1_RIGID.JPG')
  h_79_axle_1_RIGID : Subsystem
      mask Display: image('h_39_axle_1_RIGID.JPG')
  h_connector_right_angle_1_RIGID : Subsystem
      mask Display: image('connector_right_angle_1_RIGID.JPG');
  h_connector_straight_1_RIGID : Subsystem
      mask Display: image('h_connector_straight_1_RIGID.JPG')
  h_connector_straight_1_RIGID1 : Subsystem
      mask Display: image('h_connector_straight_1_RIGID.JPG')
  F : PMIOPort  Side=Left
  connections:
  Transform/LConn1 -- Transform1/LConn1 -- Transform2/LConn1 -- Transform3/LConn1 -- Transform5/LConn1 -- Transform4/LConn1
  Transform/RConn1 -- F/RConn1
  Transform1/RConn1 -- h_connector_right_angle_1_RIGID/LConn1
  Transform2/RConn1 -- h_connector_straight_1_RIGID/LConn1
  Transform3/RConn1 -- h_10_axle_1_RIGID/LConn1
  Transform4/RConn1 -- h_79_axle_1_RIGID/LConn1
  Transform5/RConn1 -- Transform6/LConn1
  Transform6/RConn1 -- h_connector_straight_1_RIGID1/LConn1

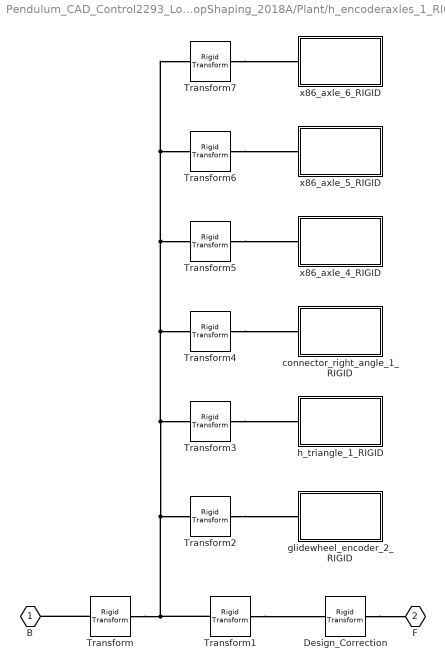
== system Pendulum_CAD_Control2293_LoopShaping_2018A/Plant/h_encoderaxles_1_RIGID ==
  Design_Correction : sm_lib/Frames and Transforms/Rigid Transform  TranslationMethod=None  TranslationStandardOffset=0  TranslationLengthUnit=mm  TranslationStandardAxis=+Z  TranslationCartesianOffset=[24.508089637866071 17.711031392187333 8.5401255470870616]  TranslationROffset=0  TranslationROffsetUnits=m  TranslationZOffset=0  TranslationZOffsetUnits=m  TranslationThetaOffset=0  TranslationThetaOffsetUnits=deg  RotationMethod=ArbitraryAxis  RotationAngleUnits=rad  RotationStandardAxis=+Z  RotationAngle=-pi/2-3.0420956054916015  RotationArbitraryAxis=[-0 0 -1]  FollAlignAxisA=+X  BaseAlignAxisA=+Y  FollAlignAxisB=+Y  BaseAlignAxisB=+Z  RotationSequenceAxes=FollowerAxes  RotationSequence=XYX  RotationSequenceAngles=[0 0 0]  RotationSequenceAnglesUnits=deg  RotationMatrix=[1 0 0; 0 1 0; 0 0 1]
  Transform : sm_lib/Frames and Transforms/Rigid Transform  TranslationMethod=Cartesian  TranslationStandardOffset=0  TranslationLengthUnit=mm  TranslationStandardAxis=+Z  TranslationCartesianOffset=[24.508089637866071 17.711031392187333 8.5401255470870616]  TranslationROffset=0  TranslationROffsetUnits=m  TranslationZOffset=0  TranslationZOffsetUnits=m  TranslationThetaOffset=0  TranslationThetaOffsetUnits=deg  RotationMethod=ArbitraryAxis  RotationAngleUnits=rad  RotationStandardAxis=+Z  RotationAngle=3.0420956054916015  RotationArbitraryAxis=[-1 1.5754106539324166e-16 -3.1641356201816969e-15]  FollAlignAxisA=+X  BaseAlignAxisA=+Y  FollAlignAxisB=+Y  BaseAlignAxisB=+Z  RotationSequenceAxes=FollowerAxes  RotationSequence=XYX  RotationSequenceAngles=[0 0 0]  RotationSequenceAnglesUnits=deg  RotationMatrix=[1 0 0; 0 1 0; 0 0 1]
  Transform1 : sm_lib/Frames and Transforms/Rigid Transform  TranslationMethod=Cartesian  TranslationStandardOffset=0  TranslationLengthUnit=mm  TranslationStandardAxis=+Z  TranslationCartesianOffset=[13.983089637865053 16.866870285554842 29.580332105627452]  TranslationROffset=0  TranslationROffsetUnits=m  TranslationZOffset=0  TranslationZOffsetUnits=m  TranslationThetaOffset=0  TranslationThetaOffsetUnits=deg  RotationMethod=ArbitraryAxis  RotationAngleUnits=rad  RotationStandardAxis=+Z  RotationAngle=2.0943951023931975  RotationArbitraryAxis=[-0.57735026918962429 -0.57735026918962629 0.57735026918962662]  FollAlignAxisA=+X  BaseAlignAxisA=+Y  FollAlignAxisB=+Y  BaseAlignAxisB=+Z  RotationSequenceAxes=FollowerAxes  RotationSequence=XYX  RotationSequenceAngles=[0 0 0]  RotationSequenceAnglesUnits=deg  RotationMatrix=[1 0 0; 0 1 0; 0 0 1]
  Transform2 : sm_lib/Frames and Transforms/Rigid Transform  TranslationMethod=Cartesian  TranslationStandardOffset=0  TranslationLengthUnit=mm  TranslationStandardAxis=+Z  TranslationCartesianOffset=[3.9830896378650893 0.057027133562839033 -3.3724154764092837]  TranslationROffset=0  TranslationROffsetUnits=m  TranslationZOffset=0  TranslationZOffsetUnits=m  TranslationThetaOffset=0  TranslationThetaOffsetUnits=deg  RotationMethod=ArbitraryAxis  RotationAngleUnits=rad  RotationStandardAxis=+Z  RotationAngle=2.152761273624384  RotationArbitraryAxis=[0.59556683818013412 0.53907354092019244 0.59556683818013556]  FollAlignAxisA=+X  BaseAlignAxisA=+Y  FollAlignAxisB=+Y  BaseAlignAxisB=+Z  RotationSequenceAxes=FollowerAxes  RotationSequence=XYX  RotationSequenceAngles=[0 0 0]  RotationSequenceAnglesUnits=deg  RotationMatrix=[1 0 0; 0 1 0; 0 0 1]
  Transform3 : sm_lib/Frames and Transforms/Rigid Transform  TranslationMethod=Cartesian  TranslationStandardOffset=0  TranslationLengthUnit=mm  TranslationStandardAxis=+Z  TranslationCartesianOffset=[88.258089637865453 17.276122100546619 25.480708592190474]  TranslationROffset=0  TranslationROffsetUnits=m  TranslationZOffset=0  TranslationZOffsetUnits=m  TranslationThetaOffset=0  TranslationThetaOffsetUnits=deg  RotationMethod=ArbitraryAxis  RotationAngleUnits=rad  RotationStandardAxis=+Z  RotationAngle=3.071252132689227  RotationArbitraryAxis=[-0.70666895787164763 -0.70666895787165263 -0.03518476888075537]  FollAlignAxisA=+X  BaseAlignAxisA=+Y  FollAlignAxisB=+Y  BaseAlignAxisB=+Z  RotationSequenceAxes=FollowerAxes  RotationSequence=XYX  RotationSequenceAngles=[0 0 0]  RotationSequenceAnglesUnits=deg  RotationMatrix=[1 0 0; 0 1 0; 0 0 1]
  Transform4 : sm_lib/Frames and Transforms/Rigid Transform  TranslationMethod=Cartesian  TranslationStandardOffset=0  TranslationLengthUnit=mm  TranslationStandardAxis=+Z  TranslationCartesianOffset=[23.258089637866103 19.749512924159973 0.70385774641775622]  TranslationROffset=0  TranslationROffsetUnits=m  TranslationZOffset=0  TranslationZOffsetUnits=m  TranslationThetaOffset=0  TranslationThetaOffsetUnits=deg  RotationMethod=ArbitraryAxis  RotationAngleUnits=rad  RotationStandardAxis=+Z  RotationAngle=3.0712521326892568  RotationArbitraryAxis=[-0.70666895787165274 -0.035184768880752892 0.70666895787164763]  FollAlignAxisA=+X  BaseAlignAxisA=+Y  FollAlignAxisB=+Y  BaseAlignAxisB=+Z  RotationSequenceAxes=FollowerAxes  RotationSequence=XYX  RotationSequenceAngles=[0 0 0]  RotationSequenceAnglesUnits=deg  RotationMatrix=[1 0 0; 0 1 0; 0 0 1]
  Transform5 : sm_lib/Frames and Transforms/Rigid Transform  TranslationMethod=Cartesian  TranslationStandardOffset=0  TranslationLengthUnit=mm  TranslationStandardAxis=+Z  TranslationCartesianOffset=[47.083089637865008 15.289827696924307 45.378138349144159]  TranslationROffset=0  TranslationROffsetUnits=m  TranslationZOffset=0  TranslationZOffsetUnits=m  TranslationThetaOffset=0  TranslationThetaOffsetUnits=deg  RotationMethod=ArbitraryAxis  RotationAngleUnits=rad  RotationStandardAxis=+Z  RotationAngle=3.1415926535897882  RotationArbitraryAxis=[2.3430246690306488e-15 -0.67106893654685129 -0.74139495709228975]  FollAlignAxisA=+X  BaseAlignAxisA=+Y  FollAlignAxisB=+Y  BaseAlignAxisB=+Z  RotationSequenceAxes=FollowerAxes  RotationSequence=XYX  RotationSequenceAngles=[0 0 0]  RotationSequenceAnglesUnits=deg  RotationMatrix=[1 0 0; 0 1 0; 0 0 1]
  Transform6 : sm_lib/Frames and Transforms/Rigid Transform  TranslationMethod=Cartesian  TranslationStandardOffset=0  TranslationLengthUnit=mm  TranslationStandardAxis=+Z  TranslationCartesianOffset=[47.083089637865342 1.032411190979611 28.000963750391605]  TranslationROffset=0  TranslationROffsetUnits=m  TranslationZOffset=0  TranslationZOffsetUnits=m  TranslationThetaOffset=0  TranslationThetaOffsetUnits=deg  RotationMethod=ArbitraryAxis  RotationAngleUnits=rad  RotationStandardAxis=+Z  RotationAngle=3.1415926535897882  RotationArbitraryAxis=[2.3430246690306472e-15 -0.67106893654685129 -0.74139495709228975]  FollAlignAxisA=+X  BaseAlignAxisA=+Y  FollAlignAxisB=+Y  BaseAlignAxisB=+Z  RotationSequenceAxes=FollowerAxes  RotationSequence=XYX  RotationSequenceAngles=[0 0 0]  RotationSequenceAnglesUnits=deg  RotationMatrix=[1 0 0; 0 1 0; 0 0 1]
  Transform7 : sm_lib/Frames and Transforms/Rigid Transform  TranslationMethod=Cartesian  TranslationStandardOffset=0  TranslationLengthUnit=mm  TranslationStandardAxis=+Z  TranslationCartesianOffset=[47.083089637864894 32.667002295676816 31.120721843199458]  TranslationROffset=0  TranslationROffsetUnits=m  TranslationZOffset=0  TranslationZOffsetUnits=m  TranslationThetaOffset=0  TranslationThetaOffsetUnits=deg  RotationMethod=ArbitraryAxis  RotationAngleUnits=rad  RotationStandardAxis=+Z  RotationAngle=3.1415926535897882  RotationArbitraryAxis=[2.3430246690306472e-15 -0.67106893654685129 -0.74139495709228975]  FollAlignAxisA=+X  BaseAlignAxisA=+Y  FollAlignAxisB=+Y  BaseAlignAxisB=+Z  RotationSequenceAxes=FollowerAxes  RotationSequence=XYX  RotationSequenceAngles=[0 0 0]  RotationSequenceAnglesUnits=deg  RotationMatrix=[1 0 0; 0 1 0; 0 0 1]
  connector_right_angle_1_RIGID : Subsystem
      mask Display: image('connector_right_angle_1_RIGID.JPG');
  glidewheel_encoder_2_RIGID : Subsystem
      mask Display: image('glidewheel_encoder_2_RIGID.JPG');
  h_triangle_1_RIGID : Subsystem
      mask Display: image('h_triangle_1_RIGID.JPG')
  x86_axle_4_RIGID : Subsystem
      mask Display: image('x86_axle_4_RIGID.JPG')
  x86_axle_5_RIGID : Subsystem
      mask Display: image('x86_axle_4_RIGID.JPG')
  x86_axle_6_RIGID : Subsystem
      mask Display: image('x86_axle_4_RIGID.JPG')
  B : PMIOPort  Side=Left
  F : PMIOPort  Port=2  Side=Right
  connections:
  Design_Correction/RConn1 -- F/RConn1
  Transform2/RConn1 -- glidewheel_encoder_2_RIGID/LConn1
  Transform3/RConn1 -- h_triangle_1_RIGID/LConn1
  Transform4/RConn1 -- connector_right_angle_1_RIGID/LConn1
  Transform5/RConn1 -- x86_axle_4_RIGID/LConn1
  Transform6/RConn1 -- x86_axle_5_RIGID/LConn1
  Transform7/RConn1 -- x86_axle_6_RIGID/LConn1
  Transform/RConn1 -- B/RConn1
  Transform/LConn1 -- Transform7/LConn1 -- Transform6/LConn1 -- Transform5/LConn1 -- Transform4/LConn1 -- Transform3/LConn1 -- Transform2/LConn1 -- Transform1/LConn1
  Transform1/RConn1 -- Design_Correction/LConn1

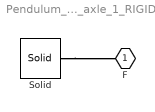
== system Pendulum_CAD_Control2293_LoopShaping_2018A/Plant/h_RIP_arm_v2_1_RIGID/h_39_axle_1_RIGID ==
  Solid : sm_lib/Body Elements/Solid  ExtGeomFileName=h_39_axle_Default_sldprt.STL  UnitType=Custom  ExtGeomFileUnits=mm  StepReaderType=HEX  ExportConvexHullGeometry=off  InertiaType=Custom  Mass=0.00052672018519800228  MassUnits=kg  CenterOfMass=[0 0 0]  CenterOfMassUnits=mm  MomentsOfInertia=[0.0012508560304239273 0.066771141817072402 0.066771141817072402]  MomentsOfInertiaUnits=kg*mm^2  ProductsOfInertia=[0 0 0]  ProductsOfInertiaUnits=kg*mm^2  BasedOnType=Density  Density=1000  DensityUnits=kg/(m^3)  DoExposeReferenceFrame=on  SerializedFrames=<Frames/>  GraphicType=FromGeometry  MarkerShape=Sphere  MarkerSize=10  MarkerSizeUnits=m  GraphicVisPropType=SimpleVisualProperties  GraphicDiffuseColor=[0.4 0.4 0.4]  GraphicSpecularColor=[0.5 0.5 0.5 1.0]  GraphicAmbientColor=[0.15 0.15 0.15 1.0]  GraphicEmissiveColor=[0.0 0.0 0.0 1.0]  GraphicShininess=75  GraphicOpacity=1  GeometryShape=FromFile
  F : PMIOPort  Side=Left
  connections:
  Solid/RConn1 -- F/RConn1

== system Pendulum_CAD_Control2293_LoopShaping_2018A/Plant/h_RIP_arm_v2_1_RIGID/h_axle_asymmetric_1_RIGID ==
  Solid : sm_lib/Body Elements/Solid  ExtGeomFileName=h_axle_asymmetric_Default_sldprt.STL  UnitType=Custom  ExtGeomFileUnits=mm  StepReaderType=HEX  ExportConvexHullGeometry=off  InertiaType=Custom  Mass=0.00086673289514495463  MassUnits=kg  CenterOfMass=[-32.724157118781108 0 0]  CenterOfMassUnits=mm  MomentsOfInertia=[0.0021064022529787255 0.30868093682298109 0.30868093682298109]  MomentsOfInertiaUnits=kg*mm^2  ProductsOfInertia=[0 0 0]  ProductsOfInertiaUnits=kg*mm^2  BasedOnType=Density  Density=1000  DensityUnits=kg/(m^3)  DoExposeReferenceFrame=on  SerializedFrames=<Frames/>  GraphicType=FromGeometry  MarkerShape=Sphere  MarkerSize=10  MarkerSizeUnits=m  GraphicVisPropType=SimpleVisualProperties  GraphicDiffuseColor=[0.4 0.4 0.4]  GraphicSpecularColor=[0.5 0.5 0.5 1.0]  GraphicAmbientColor=[0.15 0.15 0.15 1.0]  GraphicEmissiveColor=[0.0 0.0 0.0 1.0]  GraphicShininess=75  GraphicOpacity=1  GeometryShape=FromFile
  F : PMIOPort  Side=Left
  connections:
  Solid/RConn1 -- F/RConn1

== system Pendulum_CAD_Control2293_LoopShaping_2018A/Plant/h_RIP_arm_v2_1_RIGID/h_collar_1_RIGID ==
  Solid : sm_lib/Body Elements/Solid  ExtGeomFileName=h_collar_Default_sldprt.STL  UnitType=Custom  ExtGeomFileUnits=mm  StepReaderType=HEX  ExportConvexHullGeometry=off  InertiaType=Custom  Mass=0.00013195457400179582  MassUnits=kg  CenterOfMass=[-4.1099863397593017 -8.0683370661362358e-06 -1.5183618387869649e-09]  CenterOfMassUnits=mm  MomentsOfInertia=[0.00096990614842468788 0.0014236116618315936 0.0013918747546668444]  MomentsOfInertiaUnits=kg*mm^2  ProductsOfInertia=[0 0 0]  ProductsOfInertiaUnits=kg*mm^2  BasedOnType=Density  Density=1000  DensityUnits=kg/(m^3)  DoExposeReferenceFrame=on  SerializedFrames=<Frames/>  GraphicType=FromGeometry  MarkerShape=Sphere  MarkerSize=10  MarkerSizeUnits=m  GraphicVisPropType=SimpleVisualProperties  GraphicDiffuseColor=[0.4 0.4 0.4]  GraphicSpecularColor=[0.5 0.5 0.5 1.0]  GraphicAmbientColor=[0.15 0.15 0.15 1.0]  GraphicEmissiveColor=[0.0 0.0 0.0 1.0]  GraphicShininess=75  GraphicOpacity=1  GeometryShape=FromFile
  F : PMIOPort  Side=Left
  connections:
  Solid/RConn1 -- F/RConn1

== system Pendulum_CAD_Control2293_LoopShaping_2018A/Plant/h_RIP_arm_v2_1_RIGID/h_connector_straight_1_RIGID ==
  Solid : sm_lib/Body Elements/Solid  ExtGeomFileName=h_connector_straight_Default_sldprt.STL  UnitType=Custom  ExtGeomFileUnits=mm  StepReaderType=HEX  ExportConvexHullGeometry=off  InertiaType=Custom  Mass=0.00043271308549453917  MassUnits=kg  CenterOfMass=[8.0000017249971691 0 0]  CenterOfMassUnits=mm  MomentsOfInertia=[0.0031783748060293278 0.010562783552465226 0.010415546819518159]  MomentsOfInertiaUnits=kg*mm^2  ProductsOfInertia=[0 0 0]  ProductsOfInertiaUnits=kg*mm^2  BasedOnType=Density  Density=1000  DensityUnits=kg/(m^3)  DoExposeReferenceFrame=on  SerializedFrames=<Frames/>  GraphicType=FromGeometry  MarkerShape=Sphere  MarkerSize=10  MarkerSizeUnits=m  GraphicVisPropType=SimpleVisualProperties  GraphicDiffuseColor=[1 0 0]  GraphicSpecularColor=[0.5 0.5 0.5 1.0]  GraphicAmbientColor=[0.15 0.15 0.15 1.0]  GraphicEmissiveColor=[0.0 0.0 0.0 1.0]  GraphicShininess=75  GraphicOpacity=1  GeometryShape=FromFile
  F : PMIOPort  Side=Left
  connections:
  Solid/RConn1 -- F/RConn1
